simulink model "Problem5"  (R2020b)
settings: Solver=VariableStepAuto  StartTime=0.0  StopTime=10.0  RelTol=1e-3
PreLoadFcn:
  | R=10;
  | C=10e-6;
settings Model: Creator=HP  LastModifiedBy=HP

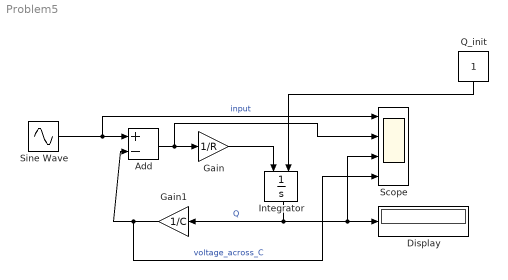
== system Problem5 ==
  Add : Sum  Inputs=+-
  Display : Display
  Gain : Gain  Gain=1/R
  Gain1 : Gain  Gain=1/C
  Integrator : Integrator  InitialConditionSource=external
  Q_init : Constant  SampleTime=-1
  Scope : Scope  NumInputPorts=4
  Sine Wave : Sin  SampleTime=0
  wires:
  Gain1/1 -> Scope/4, Add/2  "voltage_across_C"
  Sine Wave/1 -> Add/1, Scope/1  "input"
  Add/1 -> Scope/2, Gain/1
  Q_init/1 -> Integrator/2
  Integrator/1 -> Display/1, Scope/3, Gain1/1  "Q"
  Gain/1 -> Integrator/1
